simulink model "SiMappedEngine"  (R2017b)
settings: Solver=VariableStepAuto  StartTime=0.0  StopTime=inf  RelTol=1e-3  EnableMultiTasking=on
model workspace (MAT data in the model file):
  AccPwrbp = [0 1.5]
  AccSpdbp = [300 750]
  AfrStoich = 14.6
  Cps = 2
  NCyl = 4
  Pstd = 101325
  Rair = 287
  TimeCnstECP = 0.125
  TimeCnstEGR = 0.125
  TimeCnstETC = 0.085
  TimeCnstICP = 0.125
  TimeCnstIVL = 0.125
  TimeCnstMFA = 0.125
  TimeCnstSWVA = 0.125
  TimeCnstVCR = 0.125
  TimeCnstVGT = 0.15
  TimeCnstVIRL = 0.125
  TimeCnstWGA = 0.15
  Tstd = 293.15
  Vd = 0.0015
  f_air = [0 0 0 0 0 0 0 0 0 0 0 0 ... (256 elements, 16x16)]
  f_co = [0 0 0 0 0 0 0 0 0 0 0 0 ... (256 elements, 16x16)]
  f_co2 = [0 0 0 0 0 0 0 0 0 0 0 0 ... (256 elements, 16x16)]
  f_eff = [0 350.973137795 318.760126422 304.457775397 296.264860975 291.399796092 291.399634744 291.399447014 291.399182505 291.39897016 291.39870507 291.398494441 ... (256 elements, 16x16)]
  f_fuel = [0 0 0 0 0 0 0 0 0 0 0 0 ... (256 elements, 16x16)]
  f_hc = [0 0 0 0 0 0 0 0 0 0 0 0 ... (256 elements, 16x16)]
  f_nox = [0 0 0 0 0 0 0 0 0 0 0 0 ... (256 elements, 16x16)]
  f_pm = [0  0  0  0  0  0  0  0  0  0  0  0  0  0  0  0; 0  0  0  0  0  0  0  0  0  0  0  0  0  0  0  0; 0  0  0  0  0  0  0  0  0  0  0  0  0  0  0  0; 0  0  0  0  0  0  0  0  0  0  0  0  0  0  0  0; 0  0  0  0  0  0  0  0  0  0  0  0  0  0  0  0; 0  0  0  0  0  0  0  0  0  0  0  0  0  0  0  0; 0  0  0  0  0  0  0  0  0  0  0  0  0  0  0  0; 0  0  0  0  0  0  0  0  0  0  0  0  0  0  0  0; 0  0  0  0  0  0  0  0  0  0  0  0  0  0  0  0; 0  0  0  0  0  0  0  0  0  0  0  0  0  0  0  0; 0  0  0  0  0  0  0  0  0  0  0  0  0  0  0  0; 0  0  0  0  0  0  0  0  0  0  0  0  0  0  0  0; 0  0  0  0  0  0  0  0  0  0  0  0  0  0  0  0; 0  0  0  0  0  0  0  0  0  0  0  0  0  0  0  0; 0  0  0  0  0  0  0  0  0  0  0  0  0  0  0  0; 0  0  0  0  0  0  0  0  0  0  0  0  0  0  0  0]
  f_tbrake = [0 33.5982453939 45.8470209066 56.5675272071 68.244809911 76.222788533 76.2227350264 76.2228412777 76.2230443728 76.2232177986 76.223431925 76.2235956457 ... (256 elements, 16x16)]
  f_tbrake_n_bpt = [0 750 1053.57142857 1357.14285714 1660.71428571 1964.28571429 2267.85714286 2571.42857143 2875 3178.57142857 3482.14285714 3785.71428571 4089.28571429 4392.85714286 4696.42857143 5000]
  f_tbrake_t_bpt = [0 15 26.4285714286 37.8571428571 49.2857142857 60.7142857143 72.1428571429 83.5714285714 95 106.428571429 117.857142857 129.285714286 140.714285714 152.142857143 163.571428571 175]
  f_texh = [767.640829797 767.64454905 788.103208022 800.869130868 880.777600935 909.697751416 909.697090822 909.697210127 909.697674873 909.698116175 909.698671892 909.699093491 ... (256 elements, 16x16)]
  f_twc_eff_co = [0.17 0.25 0.45 0.99 0.99 0.99 0.99]
  f_twc_eff_hc = [0.21 0.375 0.75 0.98 0.98 0.98 0.98]
  f_twc_eff_lam = [0.909090909 0.944055944 0.979020979 1 1.013986014 1.048951049 1.083916084]
  f_twc_eff_nox = [0.98 0.98 0.98 0.97 0.05 0.02 0]
libraries: autolibenginesystems x1
(part 1 of 2)
settings Model: ModifiedByFormat=The MathWorks, Inc.  Creator=The MathWorks, Inc.  LastModifiedBy=The MathWorks, Inc.
settings DataIOCC: DSMLogging=off
settings CodeAppCC: StateflowObjectComments=on
settings GRTTargetCC: TargetLangStandard=C89/C90 (ANSI)
settings ConfigComp: CovMetricSettings=dsw  CovHtmlReporting=on  CovSaveCumulativeToWorkspaceVar=on  CovSaveSingleToWorkspaceVar=on  CovShowResultsExplorer=off  CovExternalEMLEnable=off
settings SimscapeCC: SimscapeNormalizeSystem=off  SimscapeNominalValues={1, 'bar'; 1, 'cm^3/s'; 1, 'bar*kg/s'; 1, 'kJ/kg'; 1, 'kW'}

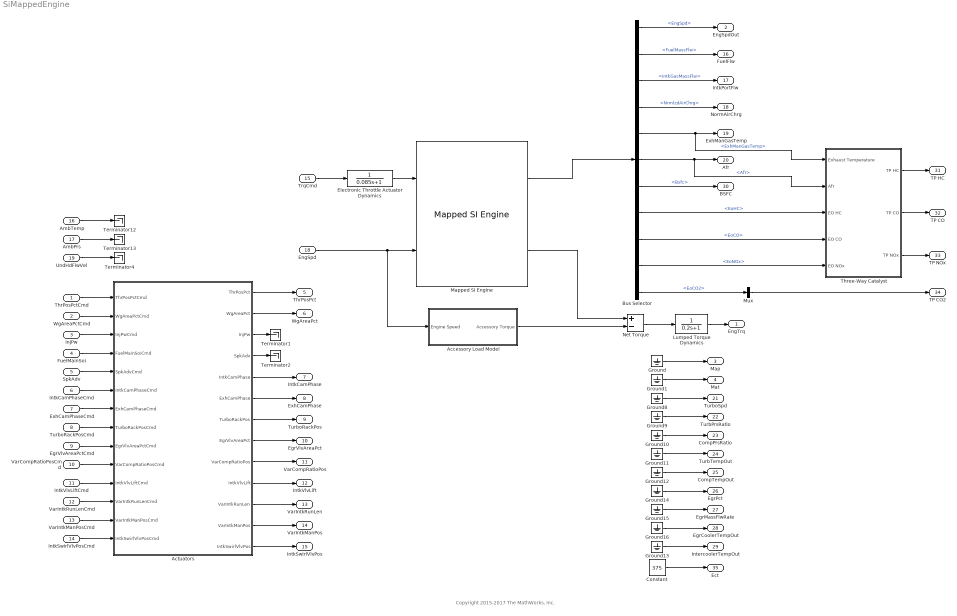
== system SiMappedEngine ==
  note: Copyright 2015-2017 The MathWorks, Inc.
  ThrPosPctCmd : Inport
  WgAreaPctCmd : Inport  Port=2
  InjPw : Inport  Port=3
  FuelMainSoi : Inport  Port=4
  SpkAdv : Inport  Port=5
  IntkCamPhaseCmd : Inport  Port=6
  ExhCamPhaseCmd : Inport  Port=7
  TurboRackPosCmd : Inport  Port=8
  EgrVlvAreaPctCmd : Inport  Port=9
  VarCompRatioPosCmd : Inport  Port=10
  IntkVlvLiftCmd : Inport  Port=11
  VarIntkRunLenCmd : Inport  Port=12
  VarIntkManPosCmd : Inport  Port=13
  IntkSwirlVlvPosCmd : Inport  Port=14
  TrqCmd : Inport  Port=15  Unit=N*m
  AmbTemp : Inport  Port=16  Unit=K
  AmbPrs : Inport  Port=17  Unit=Pa
  EngSpd : Inport  Port=18  Interpolate=off
  UndHdFlwVel : Inport  Port=19  Unit=m/s
  Accessory Load Model : Subsystem
  Actuators : Subsystem
  Bus Selector : BusSelector  OutputSignals=EngSpd,FuelMassFlw,IntkGasMassFlw,NrmlzdAirChrg,ExhManGasTemp,Afr,Bsfc,EoHC,EoCO,EoNOx,EoCO2
  Constant : Constant  Value=375
  Electronic Throttle Actuator Dynamics : TransferFcn  Denominator=[0.085 1]
  Ground{,1,8..16} (11 alike) : Ground
  Lumped Torque Dynamics : TransferFcn  Denominator=[0.2 1]
  Mapped SI Engine : autolibenginesystems/Mapped SI Engine  TurboLagCheckbox=off  rowVarName=TrqCmd  f_tbrake_t_bpt=f_tbrake_t_bpt  colVarName=EngSpd  f_tbrake_n_bpt=f_tbrake_n_bpt  NCyl=NCyl  Cps=Cps  Vd=Vd  Rair=Rair  Pstd=Pstd  Tstd=Tstd  Use1=on  Use2=on  Use3=on  Use4=on  Use5=on  Use6=on  Use7=on  Use8=on  Use9=on  Use10=off  f_tbrake_bst=[0, 79.51 81.38 91.45 97.78 102.6 106.2 109.6 111.6 113.4 113.9 113.3 115 111.9 108.1 105]  tau_thr=0.2  tau_bst_rising=1.5  tau_bst_falling=1  tq_blend_frac=0.01  Name1=Brake Torque  f_tbrake=f_tbrake  Name2=Air Mass Flow  f_air=f_air  Name3=Fuel Flow  f_fuel=f_fuel  Name4=Exhaust Temperature  f_texh=f_texh  Name5=[514.035834811904 472.420001567292 468.560027988283 467.25113080026 469.376552017678 472.466817198703 477.085817372135 482.089315297269 488.091390331625 495.511698221518 503.603605470575 513.545560314063 524.708632042863 537.901582788691 547.57773149968;372.215126833557 362.023004934345 357.061196096605 354.397690627091 353.695017513094 355.069365264177 357.083429546077 359.150328797338 361.216056662124 363.787443052002 368.052362907894 373.273609540704 379.492527390704 387.062712835118 392.829054841793;326.61409907784 316.864439849348 311.950172215081 309.623392513349 308.520317680707 308.639621388036 309.473192508284 311.206605049837 312.435624355117 314.372691523229 315.240918825382 319.20290576235 323.194337587902 328.582300779183 332.542719046893;302.302708332089 292.988583490457 288.191388571794 286.11397076702 285.309041994516 284.733243126823 284.189019193475 282.574319206257 284.12037910983 287.79556805798 288.17907837576 290.209859138972 293.679673638155 297.45343144841 300.726288347892;288.700928736811 278.551672830084 273.400833959319 270.536547804349 267.833435583205 267.119414364878 265.972950018046 266.740920363958 268.048224971445 270.838385340352 270.778373480454 272.970259132319 275.506872347887 278.72040783414 281.813869092965;284.845821006168 269.394829178651 263.982926589081 260.478586413209 257.028965789929 255.931084916756 255.874470882376 256.430426703396 258.42024291946 257.808327020541 258.950655075076 261.079050323518 263.461085730423 266.38231289239 269.295763051135;288.386442360439 264.344752526028 257.213462364171 254.168296127581 250.527881300837 249.049345022729 250.073316495023 249.665324624047 248.602086912424 249.355944667699 250.714426186754 252.515083416491 254.990022645247 258.139224389126 258.88586921331;288.386442360439 267.197275532715 251.193959608514 247.553061326459 246.301141111655 244.695607301207 242.621990784403 242.304630618562 242.866111727694 243.758994026591 244.970247326866 246.821991594926 249.775586923996 251.245282116681 253.478417008787;288.386442360439 277.668290802935 252.854894387889 243.851167532952 241.861572413297 238.689990387976 238.067198500515 238.072941982365 238.685701547209 239.312989651019 240.673403883432 242.669277941474 245.301951037108 246.789302536782 247.789414843363;288.386442360439 277.504945286633 270.702819258252 245.731480615597 238.395305310031 236.119281963407 235.324944828075 235.181758472016 235.88354482046 236.67974458838 237.758701429304 239.923633193373 242.123394230695 242.998011528535 244.273734537053;288.386442360439 277.504945286633 279.349376222353 263.18046263446 241.569205761561 235.781254475789 234.445285156959 234.881842747232 234.822376790859 235.79445272942 237.439515459863 239.43946089678 241.356663529347 242.334213324245 244.486434215002;288.386442360439 277.504945286633 279.349376222353 299.505188255346 260.338046997911 239.40420517855 235.256510952508 234.880694514868 234.31593804329 236.319225658558 237.102712721133 239.012709272806 240.75776355138 241.336977805019 256.331160738088;288.386442360439 277.504945286633 279.349376222353 299.505188255346 320.026630425816 342.9283130372 241.52452305243 328.315966517739 244.549289572305 251.858270967766 240.732881082116 242.07382019702 244.535478307747 249.496579565711 263.930188372987;288.386442360439 277.504945286633 279.349376222353 299.505188255346 320.026630425816 342.9283130372 345.883623776508 328.315966517739 317.337354078743 314.624789096503 254.725548546873 250.384805432702 271.371327381584 265.474840242786 277.521724347837;288.386442360439 277.504945286633 279.349376222353 299.505188255346 320.026630425816 342.9283130372 345.883623776508 328.315966517739 319.749039003082 318.879022253509 311.782458169383 312.350604651759 319.747883103035 320.841917879101 308.256263223954]  f_eff=f_eff  Name6=EO HC  f_hc=f_hc  Name7=EO CO  f_co=f_co  Name8=EO NOx  f_nox=f_nox  Name9=EO CO2  f_co2=f_co2  Name10=Brake Torque  f_pm=f_pm
      settings: SourceProductName=Powertrain Blockset  SourceProductBaseCode=PW
  Mux : Mux  Inputs=1
  Net Torque : Sum  Inputs=+-
  Terminator{1..2,4,12..13} (5 alike) : Terminator
  Three-Way Catalyst : Subsystem
  EngTrq : Outport  Unit=N*m
  EngSpdOut : Outport  Port=2
  Map : Outport  Port=3  Unit=Pa
  Mat : Outport  Port=4  Unit=K
  ThrPosPct : Outport  Port=5
  WgAreaPct : Outport  Port=6
  IntkCamPhase : Outport  Port=7
  ExhCamPhase : Outport  Port=8
  TurboRackPos : Outport  Port=9
  EgrVlvAreaPct : Outport  Port=10
  VarCompRatioPos : Outport  Port=11
  IntkVlvLift : Outport  Port=12
  VarIntkRunLen : Outport  Port=13
  VarIntkManPos : Outport  Port=14
  IntkSwirlVlvPos : Outport  Port=15
  FuelFlw : Outport  Port=16
  IntkPortFlw : Outport  Port=17
  NormAirChrg : Outport  Port=18
  ExhManGasTemp : Outport  Port=19
  Afr : Outport  Port=20  Unit=1
  TurboSpd : Outport  Port=21  Unit=rad/s
  TurbPrsRatio : Outport  Port=22  Unit=1
  CompPrsRatio : Outport  Port=23  Unit=1
  TurbTempOut : Outport  Port=24  Unit=K
  CompTempOut : Outport  Port=25  Unit=K
  EgrPct : Outport  Port=26  Unit=%
  EgrMassFlwRate : Outport  Port=27  Unit=kg/s
  EgrCoolerTempOut : Outport  Port=28  Unit=K
  IntercoolerTempOut : Outport  Port=29  Unit=K
  BSFC : Outport  Port=30
  TP HC : Outport  Port=31
  TP CO : Outport  Port=32
  TP NOx : Outport  Port=33
  TP CO2 : Outport  Port=34
  Ect : Outport  Port=35  Unit=K
  wires:
  Mapped SI Engine/1 -> Bus Selector/1
  Bus Selector/5 -> Three-Way Catalyst/1(Exhaust Temperature), ExhManGasTemp/1  "<ExhManGasTemp>"
  Bus Selector/6 -> Three-Way Catalyst/2(Afr), Afr/1  "<Afr>"
  EngSpd/1 -> Accessory Load Model/1(Engine Speed), Mapped SI Engine/2
  Accessory Load Model/1(Accessory Torque) -> Net Torque/2
  Lumped Torque Dynamics/1 -> EngTrq/1
  Bus Selector/1 -> EngSpdOut/1  "<EngSpd>"
  Bus Selector/2 -> FuelFlw/1  "<FuelMassFlw>"
  Bus Selector/3 -> IntkPortFlw/1  "<IntkGasMassFlw>"
  Bus Selector/8 -> Three-Way Catalyst/3(EO HC)  "<EoHC>"
  Bus Selector/9 -> Three-Way Catalyst/4(EO CO)  "<EoCO>"
  Bus Selector/10 -> Three-Way Catalyst/5(EO NOx)  "<EoNOx>"
  Bus Selector/11 -> Mux/1  "<EoCO2>"
  Three-Way Catalyst/1(TP HC) -> TP HC/1
  Three-Way Catalyst/2(TP CO) -> TP CO/1
  Three-Way Catalyst/3(TP NOx) -> TP NOx/1
  Mux/1 -> TP CO2/1
  TrqCmd/1 -> Electronic Throttle Actuator Dynamics/1
  Net Torque/1 -> Lumped Torque Dynamics/1
  Bus Selector/7 -> BSFC/1  "<Bsfc>"
  Bus Selector/4 -> NormAirChrg/1  "<NrmlzdAirChrg>"
  Mapped SI Engine/2 -> Net Torque/1
  Electronic Throttle Actuator Dynamics/1 -> Mapped SI Engine/1
  IntkCamPhaseCmd/1 -> Actuators/6(IntkCamPhaseCmd)
  Ground16/1 -> EgrCoolerTempOut/1
  Ground14/1 -> EgrPct/1
  Ground13/1 -> IntercoolerTempOut/1
  Ground12/1 -> CompTempOut/1
  FuelMainSoi/1 -> Actuators/4(FuelMainSoiCmd)
  EgrVlvAreaPctCmd/1 -> Actuators/9(EgrVlvAreaPctCmd)
  Ground11/1 -> TurbTempOut/1
  ExhCamPhaseCmd/1 -> Actuators/7(ExhCamPhaseCmd)
  Ground9/1 -> TurbPrsRatio/1
  Ground8/1 -> TurboSpd/1
  SpkAdv/1 -> Actuators/5(SpkAdvCmd)
  AmbTemp/1 -> Terminator12/1
  Ground15/1 -> EgrMassFlwRate/1
  TurboRackPosCmd/1 -> Actuators/8(TurboRackPosCmd)
  ThrPosPctCmd/1 -> Actuators/1(ThrPosPctCmd)
  WgAreaPctCmd/1 -> Actuators/2(WgAreaPctCmd)
  InjPw/1 -> Actuators/3(InjPwCmd)
  Ground10/1 -> CompPrsRatio/1
  Ground1/1 -> Mat/1
  Ground/1 -> Map/1
  AmbPrs/1 -> Terminator13/1
  IntkVlvLiftCmd/1 -> Actuators/11(IntkVlvLiftCmd)
  VarCompRatioPosCmd/1 -> Actuators/10(VarCompRatioPosCmd)
  VarIntkRunLenCmd/1 -> Actuators/12(VarIntkRunLenCmd)
  IntkSwirlVlvPosCmd/1 -> Actuators/14(IntkSwirlVlvPosCmd)
  VarIntkManPosCmd/1 -> Actuators/13(VarIntkManPosCmd)
  UndHdFlwVel/1 -> Terminator4/1
  Actuators/1(ThrPosPct) -> ThrPosPct/1
  Actuators/2(WgAreaPct) -> WgAreaPct/1
  Actuators/3(InjPw) -> Terminator1/1
  Actuators/4(SpkAdv) -> Terminator2/1
  Actuators/5(IntkCamPhase) -> IntkCamPhase/1
  Actuators/6(ExhCamPhase) -> ExhCamPhase/1
  Actuators/7(TurboRackPos) -> TurboRackPos/1
  Actuators/8(EgrVlvAreaPct) -> EgrVlvAreaPct/1
  Actuators/9(VarCompRatioPos) -> VarCompRatioPos/1
  Actuators/10(IntkVlvLift) -> IntkVlvLift/1
  Actuators/11(VarIntkRunLen) -> VarIntkRunLen/1
  Actuators/12(VarIntkManPos) -> VarIntkManPos/1
  Actuators/13(IntkSwirlVlvPos) -> IntkSwirlVlvPos/1
  Constant/1 -> Ect/1
